simulink model "tpauto7pasfini"  (R2019a)
settings: Solver=VariableStepAuto  StartTime=0.0  StopTime=10.0  RelTol=1e-3
settings Model: Creator=mbenahme  LastModifiedBy=mbenahme

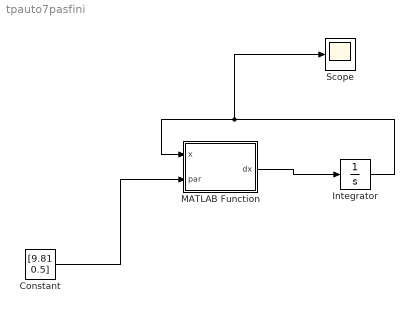
== system tpauto7pasfini ==
  Constant : Constant  Value=[9.81 0.5]
  Integrator : Integrator  InitialCondition=pi/4
  MATLAB Function : MATLAB Function  TreatAsAtomicUnit=on
  Scope : Scope
  wires:
  Constant/1 -> MATLAB Function/2(par)
  MATLAB Function/1(dx) -> Integrator/1
  Integrator/1 -> Scope/1, MATLAB Function/1(x)

== matlab function tpauto7pasfini/MATLAB Function ==
  data: x input; dx output; par input
function dx = fcn(x, par)

dx = [x(2);(par(1)/par(2))*sin(x(1))];
